simulink model "Question_2"  (R2024b)
settings: Solver=VariableStepAuto  StartTime=0.0  StopTime=10.0  RelTol=1e-3
model workspace (MAT data in the model file):
  F = 100
  M = 200
  k = 10
settings Model: Creator=Sagar  LastModifiedBy=Sagar

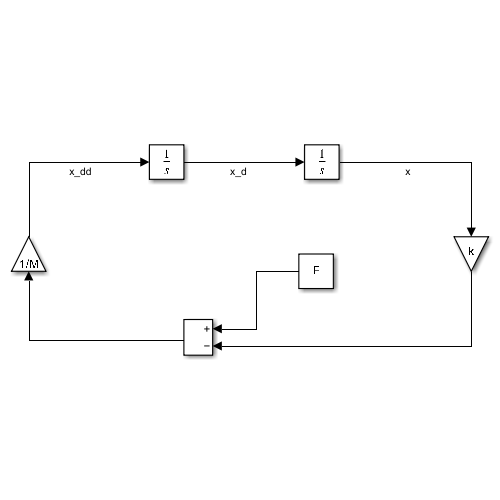
[thumbnail: Simulink's stored preview of the top-level diagram]
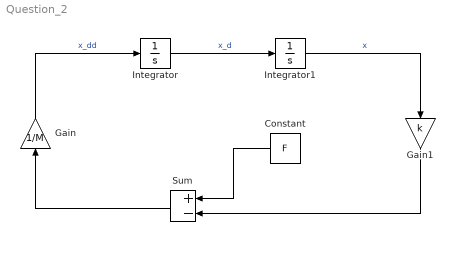
== system Question_2 ==
  Constant : Constant  Value=F
  Gain : Gain  Gain=1/M
  Gain1 : Gain  Gain=k
  Integrator : Integrator
  Integrator1 : Integrator
  Sum : Sum  Inputs=+-
  wires:
  Integrator/1 -> Integrator1/1  "x_d"
  Gain/1 -> Integrator/1  "x_dd"
  Integrator1/1 -> Gain1/1  "x"
  Gain1/1 -> Sum/2
  Sum/1 -> Gain/1
  Constant/1 -> Sum/1
